simulink subsystem "dc_motor_transfer"  (R2019b)
settings: Solver=VariableStepAuto  StartTime=0.0  StopTime=10.0  RelTol=1e-3
undefined symbols (not defined in the file): b, J, k_e, k_m, L, R
settings Model: Creator=isakaslund  LastModifiedBy=isakaslund

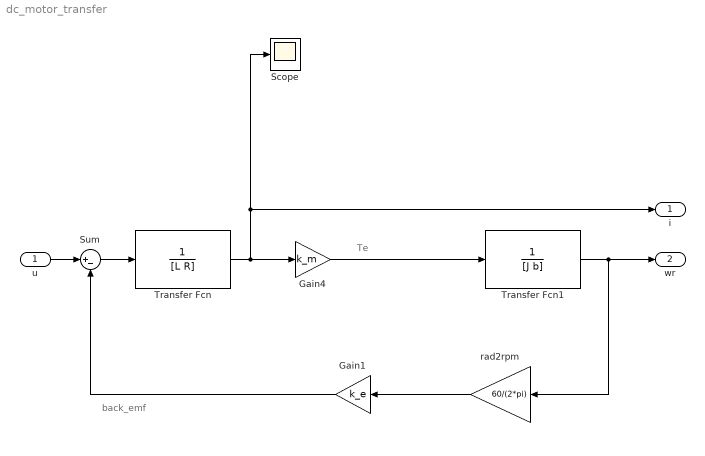
== system dc_motor_transfer ==
  note: back_emf
  note: Te
  u : Inport
  Gain1 : Gain  Gain=k_e
  Gain4 : Gain  Gain=k_m
  Scope : Scope
  Sum : Sum  Inputs=|+-
  Transfer Fcn : TransferFcn  Denominator=[L R]
  Transfer Fcn1 : TransferFcn  Denominator=[J b]
  rad2rpm : Gain  Gain=60/(2*pi)
  i : Outport  VectorParamsAs1DForOutWhenUnconnected=off
  "wr " : Outport  Port=2  VectorParamsAs1DForOutWhenUnconnected=off
  wires:
  Transfer Fcn/1 -> Scope/1, i/1, Gain4/1
  Gain4/1 -> Transfer Fcn1/1
  Transfer Fcn1/1 -> "wr "/1, rad2rpm/1
  Sum/1 -> Transfer Fcn/1
  u/1 -> Sum/1
  Gain1/1 -> Sum/2
  rad2rpm/1 -> Gain1/1
